simulink model "SS"  (R2022b)
settings: Solver=VariableStepAuto  StartTime=0.0  StopTime=10.0  RelTol=1e-3
undefined symbols (not defined in the file): degs2rpm, der, DiscIntNeverNeededParam, drv, gbox, K, mld, mot, Nu, Nx, sens, simul
settings Model: Creator=emanuelevitetta  LastModifiedBy=emanuelevitetta

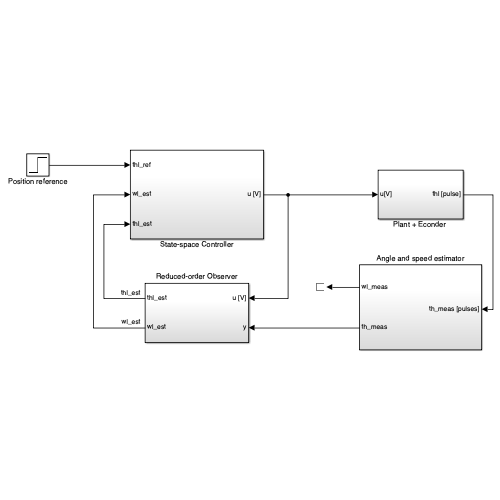
[thumbnail: Simulink's stored preview of the top-level diagram]
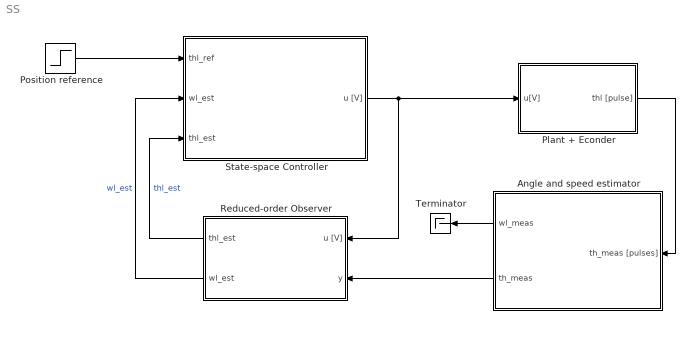
== system SS ==
  Angle and speed estimator : Subsystem
  "Plant + Econder " : Subsystem
  Position reference : Step
  Reduced-order Observer : Subsystem
  State-space Controller : Subsystem
  Terminator : Terminator
  wires:
  "Plant + Econder "/1(thl [pulse]) -> Angle and speed estimator/1(th_meas [pulses])
  Position reference/1 -> State-space Controller/1("thl_ref ")
  Reduced-order Observer/2(wl_est) -> State-space Controller/2(wl_est)  "wl_est"
  State-space Controller/1(u [V]) -> "Plant + Econder "/1(u[V]), Reduced-order Observer/1(u [V])
  Reduced-order Observer/1("thl_est ") -> State-space Controller/3(thl_est)  "thl_est"
  Angle and speed estimator/2(th_meas) -> Reduced-order Observer/2(y)
  Angle and speed estimator/1(wl_meas) -> Terminator/1

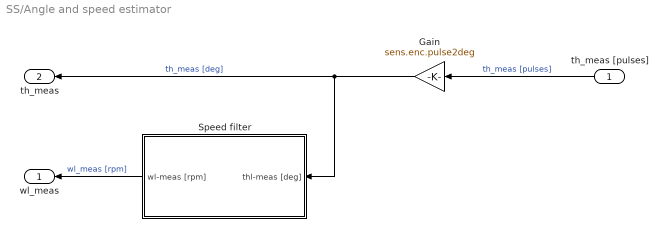
== system SS/Angle and speed estimator ==
  th_meas [pulses] : Inport
  Gain : Gain  Gain=sens.enc.pulse2deg
  Speed filter : Subsystem
  wl_meas : Outport
  th_meas : Outport  Port=2
  wires:
  Speed filter/1(wl-meas [rpm]) -> wl_meas/1  "wl_meas [rpm]"
  th_meas [pulses]/1 -> Gain/1  "th_meas [pulses]"
  Gain/1 -> Speed filter/1(thl-meas [deg]), th_meas/1  "th_meas [deg]"

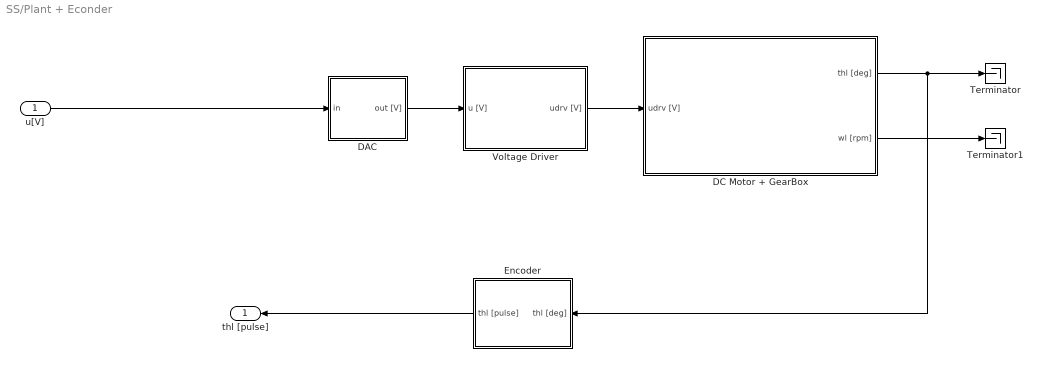
== system SS/Plant + Econder  ==
  u[V] : Inport
  DAC : Subsystem
  DC Motor + GearBox : Subsystem
  Encoder : Subsystem
  Terminator : Terminator
  Terminator1 : Terminator
  Voltage Driver : Subsystem
  thl [pulse] : Outport
  wires:
  DC Motor + GearBox/1(thl [deg]) -> Encoder/1(thl [deg]), Terminator/1
  DC Motor + GearBox/2(wl [rpm]) -> Terminator1/1
  Voltage Driver/1(udrv [V]) -> DC Motor + GearBox/1(udrv [V])
  u[V]/1 -> DAC/1(in)
  DAC/1(out [V]) -> Voltage Driver/1(u [V])
  Encoder/1(thl [pulse]) -> thl [pulse]/1

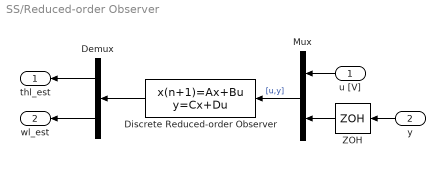
== system SS/Reduced-order Observer ==
  u [V] : Inport
  y : Inport  Port=2
  Demux : Demux  Outputs=2
  Discrete Reduced-order Observer : DiscreteStateSpace
  Mux : Mux  Inputs=2
  ZOH : ZeroOrderHold
  "thl_est " : Outport
  wl_est : Outport  Port=2
  wires:
  Mux/1 -> Discrete Reduced-order Observer/1  "[u,y]"
  u [V]/1 -> Mux/1
  Discrete Reduced-order Observer/1 -> Demux/1
  ZOH/1 -> Mux/2
  y/1 -> ZOH/1
  Demux/1 -> "thl_est "/1
  Demux/2 -> wl_est/1

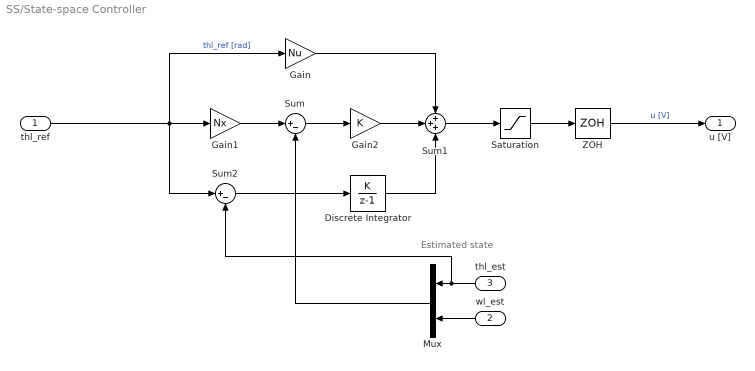
== system SS/State-space Controller ==
  note: Estimated state
  "thl_ref " : Inport
  wl_est : Inport  Port=2
  thl_est : Inport  Port=3
  Discrete Integrator : DiscreteIntegrator  IntegratorMethod=Accumulation: Forward Euler  ICPrevOutput=DiscIntNeverNeededParam  ICPrevScaledInput=DiscIntNeverNeededParam
  Gain : Gain  Gain=Nu
  Gain1 : Gain  Gain=Nx
  Gain2 : Gain  Gain=K
  Mux : Mux  Inputs=2
  Saturation : Saturate  UpperLimit=10  LowerLimit=-10
  Sum : Sum  Inputs=|+-
  Sum1 : Sum  Inputs=+++
  Sum2 : Sum  Inputs=|+-
  ZOH : ZeroOrderHold
  u [V] : Outport
  wires:
  Mux/1 -> Sum/2
  "thl_ref "/1 -> Gain1/1, Gain/1, Sum2/1  "thl_ref [rad]"
  Gain1/1 -> Sum/1
  Sum/1 -> Gain2/1
  Gain2/1 -> Sum1/2
  Sum1/1 -> Saturation/1
  Gain/1 -> Sum1/1
  Sum2/1 -> Discrete Integrator/1
  Discrete Integrator/1 -> Sum1/3
  Saturation/1 -> ZOH/1
  ZOH/1 -> u [V]/1  "u [V]"
  thl_est/1 -> Sum2/2, Mux/1
  wl_est/1 -> Mux/2

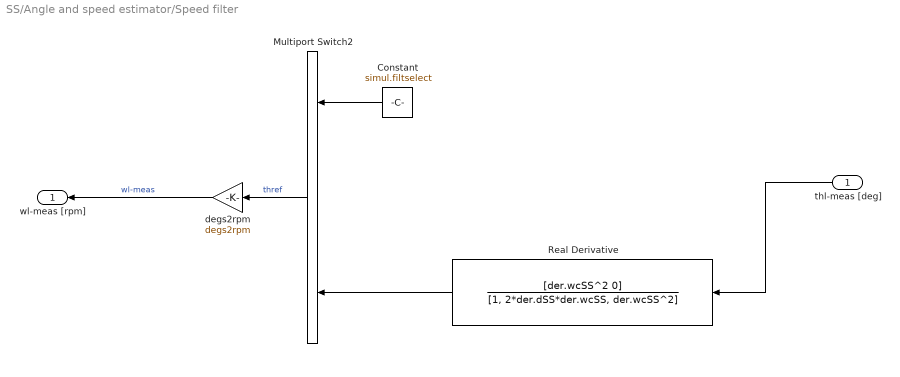
== system SS/Angle and speed estimator/Speed filter ==
  thl-meas [deg] : Inport
  Constant : Constant  Value=simul.filtselect
  Multiport Switch2 : MultiPortSwitch  Inputs=2  SaturateOnIntegerOverflow=off  InputSameDT=off
  Real Derivative : TransferFcn  Numerator=[der.wcSS^2 0]  Denominator=[1, 2*der.dSS*der.wcSS, der.wcSS^2]
  degs2rpm : Gain  Gain=degs2rpm
  wl-meas [rpm] : Outport
  wires:
  degs2rpm/1 -> wl-meas [rpm]/1  "wl-meas"
  Real Derivative/1 -> Multiport Switch2/3
  Multiport Switch2/1 -> degs2rpm/1  "thref"
  Constant/1 -> Multiport Switch2/1
  thl-meas [deg]/1 -> Real Derivative/1

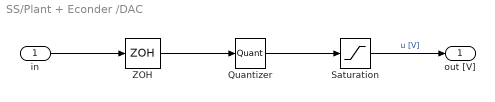
== system SS/Plant + Econder /DAC ==
  in : Inport
  Quantizer : Quantizer  QuantizationInterval=1
  Saturation : Saturate  UpperLimit=10  LowerLimit=-10
  ZOH : ZeroOrderHold  SampleTime=0.001
  out [V] : Outport
  wires:
  Saturation/1 -> out [V]/1  "u [V]"
  in/1 -> ZOH/1
  ZOH/1 -> Quantizer/1
  Quantizer/1 -> Saturation/1

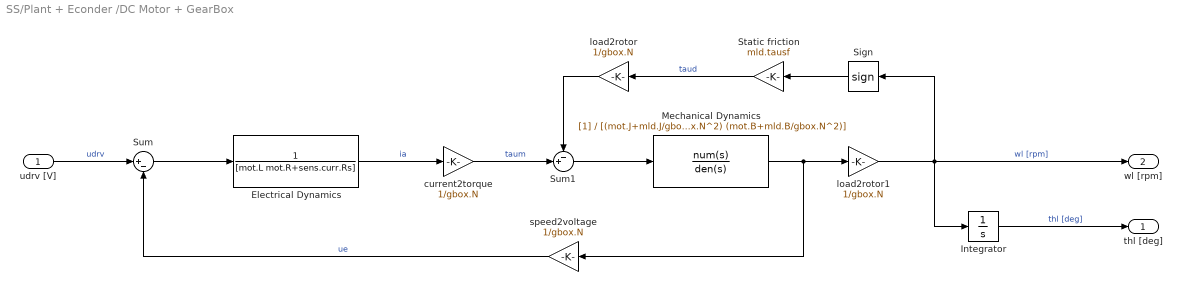
== system SS/Plant + Econder /DC Motor + GearBox ==
  udrv [V] : Inport
  Electrical Dynamics : TransferFcn  Denominator=[mot.L mot.R+sens.curr.Rs]
  Integrator : Integrator
  Mechanical Dynamics : TransferFcn  Denominator=[(mot.J+mld.J/gbox.N^2) (mot.B+mld.B/gbox.N^2)]
  Sign : Signum  ZeroCross=off
  Static friction : Gain  Gain=mld.tausf
  Sum : Sum  Inputs=|+-
  Sum1 : Sum  Inputs=-+|
  current2torque : Gain  Gain=1/gbox.N
  load2rotor : Gain  Gain=1/gbox.N
  load2rotor1 : Gain  Gain=1/gbox.N
  speed2voltage : Gain  Gain=1/gbox.N
  thl [deg] : Outport
  wl [rpm] : Outport  Port=2
  wires:
  load2rotor1/1 -> Integrator/1, wl [rpm]/1, Sign/1  "wl [rpm]"
  Sign/1 -> Static friction/1
  Electrical Dynamics/1 -> current2torque/1  "ia"
  Sum1/1 -> Mechanical Dynamics/1
  Integrator/1 -> thl [deg]/1  "thl [deg]"
  load2rotor/1 -> Sum1/1
  udrv [V]/1 -> Sum/1  "udrv"
  current2torque/1 -> Sum1/2  "taum"
  Static friction/1 -> load2rotor/1  "taud"
  speed2voltage/1 -> Sum/2  "ue"
  Sum/1 -> Electrical Dynamics/1
  Mechanical Dynamics/1 -> speed2voltage/1, load2rotor1/1

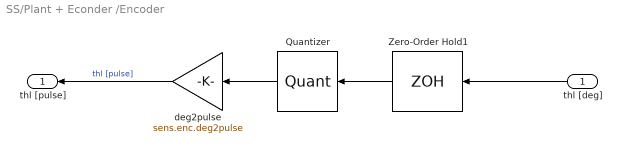
== system SS/Plant + Econder /Encoder ==
  thl [deg] : Inport
  Quantizer : Quantizer  QuantizationInterval=sens.enc.pulse2deg
  Zero-Order Hold1 : ZeroOrderHold  SampleTime=0.001
  deg2pulse : Gain  Gain=sens.enc.deg2pulse
  thl [pulse] : Outport
  wires:
  thl [deg]/1 -> Zero-Order Hold1/1
  Zero-Order Hold1/1 -> Quantizer/1
  deg2pulse/1 -> thl [pulse]/1  "thl [pulse]"
  Quantizer/1 -> deg2pulse/1

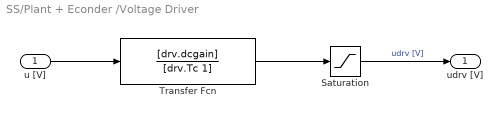
== system SS/Plant + Econder /Voltage Driver ==
  u [V] : Inport
  Saturation : Saturate  UpperLimit=12  LowerLimit=-12
  Transfer Fcn : TransferFcn  Numerator=[drv.dcgain]  Denominator=[drv.Tc 1]
  udrv [V] : Outport
  wires:
  Saturation/1 -> udrv [V]/1  "udrv [V]"
  u [V]/1 -> Transfer Fcn/1
  Transfer Fcn/1 -> Saturation/1
